simulink model "UserSteerTorque"  (Simulink 7.5)
settings: Solver=ode45  StartTime=0.0  StopTime=inf  RelTol=1e-3
libraries: CarMaker4SL x4, simulink x1
(part 2 of 2)

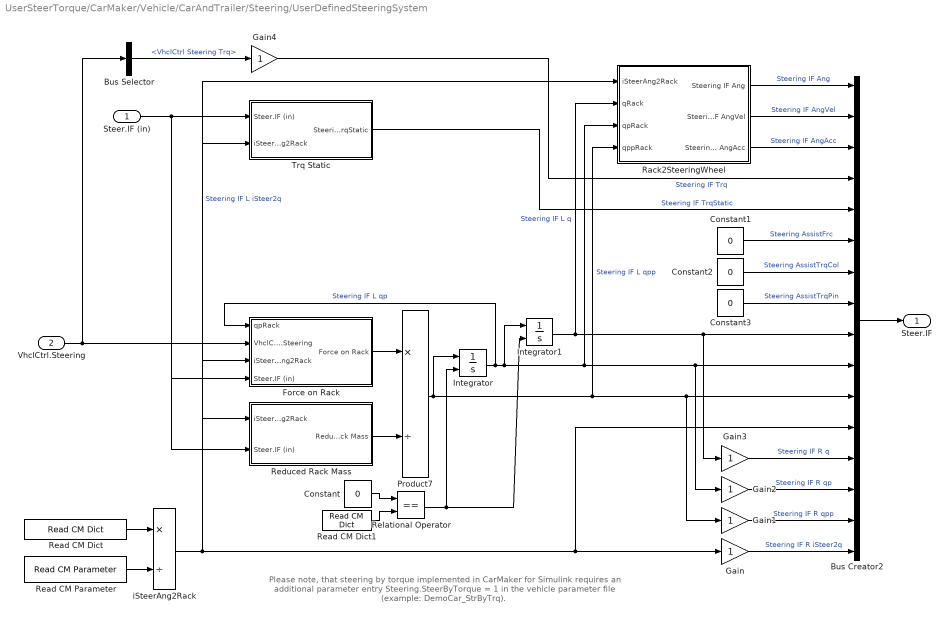
== system UserSteerTorque/CarMaker/Vehicle/CarAndTrailer/Steering/UserDefinedSteeringSystem ==
  note: Please note, that steering by torque implemented in
      | CarMaker for Simulink requires an additional parameter entry
      | Steering.SteerByTorque = 1
      | in the vehicle parameter file (example: DemoCar_StrByTrq).
  Steer.IF (in) : Inport  OutDataType=sfix(16)  OutScaling=2^0
  VhclCtrl.Steering : Inport  Port=2  OutDataType=sfix(16)  OutScaling=2^0
  Bus Creator2 : BusCreator  Inputs=16
  Bus Selector : BusSelector  OutputSignals=VhclCtrl Steering Trq
  Constant{,1..3} (4 alike) : Constant  Value=0  OutDataType=sfix(16)  OutScaling=2^0
  Force on Rack : Subsystem
  Gain{,1..4} (5 alike) : Gain  ParameterDataType=sfix(16)  ParameterScaling=2^0  OutDataType=sfix(16)  OutScaling=2^0
  Integrator : Integrator  ExternalReset=level
  Integrator1 : Integrator  ExternalReset=level
  Product7 : Product  Inputs=*/  OutDataType=sfix(16)  OutScaling=2^0  SaturateOnIntegerOverflow=on  InputSameDT=on  OutDataTypeStr=Inherit: Same as first input
  Rack2SteeringWheel : Subsystem
  Read CM Dict : CarMaker4SL/Read CM Dict  xname=Steer.Cfg.PosSign  xsync=off
  Read CM Dict1 : CarMaker4SL/Read CM Dict  xname=Time  xsync=off
  Read CM Parameter : CarMaker4SL/Read CM Parameter  xfile=Steering  xkey=Steering.Rack2StWhl  xnout=1  xdefaults=[]  xmuxed=off
  Reduced Rack Mass : Subsystem
  Relational Operator : RelationalOperator  Operator===
  Trq Static : Subsystem
  iSteerAng2Rack : Product  Inputs=*/  OutDataType=sfix(16)  OutScaling=2^0  SaturateOnIntegerOverflow=on  InputSameDT=on  OutDataTypeStr=Inherit: Same as first input
  Steer.IF : Outport  OutDataType=sfix(16)  OutScaling=2^0
  wires:
  Bus Selector/1 -> Gain4/1  "<VhclCtrl Steering Trq>"
  Gain4/1 -> Bus Creator2/4  "Steering IF Trq"
  Gain3/1 -> Bus Creator2/13  "Steering IF R q"
  Gain2/1 -> Bus Creator2/14  "Steering IF R qp"
  Gain1/1 -> Bus Creator2/15  "Steering IF R qpp"
  Gain/1 -> Bus Creator2/16  "Steering IF R iSteer2q"
  Read CM Dict/1 -> iSteerAng2Rack/1
  Read CM Parameter/1 -> iSteerAng2Rack/2
  Steer.IF (in)/1 -> Trq Static/1(Steer.IF (in)), Force on Rack/4(Steer.IF (in)), Reduced Rack Mass/2(Steer.IF (in))
  Force on Rack/1(Force on Rack) -> Product7/1
  Reduced Rack Mass/1(Reduced Rack Mass) -> Product7/2
  iSteerAng2Rack/1 -> Rack2SteeringWheel/1(iSteerAng2Rack), Trq Static/2(iSteerAng2Rack), Force on Rack/3(iSteerAng2Rack), Reduced Rack Mass/1(iSteerAng2Rack), Gain/1, Bus Creator2/12  "Steering IF L iSteer2q"
  Integrator1/1 -> Rack2SteeringWheel/2(qRack), Gain3/1, Bus Creator2/9  "Steering IF L q"
  Trq Static/1(Steering IF TrqStatic) -> Bus Creator2/5  "Steering IF TrqStatic"
  Rack2SteeringWheel/1(Steering IF Ang) -> Bus Creator2/1  "Steering IF Ang"
  Rack2SteeringWheel/2(Steering IF AngVel) -> Bus Creator2/2  "Steering IF AngVel"
  Rack2SteeringWheel/3(Steering IF AngAcc) -> Bus Creator2/3  "Steering IF AngAcc"
  VhclCtrl.Steering/1 -> Bus Selector/1, Force on Rack/2(VhclCtrl.Steering)
  Integrator/1 -> Force on Rack/1(qpRack), Rack2SteeringWheel/3(qpRack), Gain2/1, Bus Creator2/10, Integrator1/1  "Steering IF L qp"
  Product7/1 -> Rack2SteeringWheel/4(qppRack), Gain1/1, Bus Creator2/11, Integrator/1  "Steering IF L qpp"
  Relational Operator/1 -> Integrator/2, Integrator1/2
  Read CM Dict1/1 -> Relational Operator/2
  Constant/1 -> Relational Operator/1
  Bus Creator2/1 -> Steer.IF/1
  Constant1/1 -> Bus Creator2/6  "Steering AssistFrc"
  Constant2/1 -> Bus Creator2/7  "Steering AssistTrqCol"
  Constant3/1 -> Bus Creator2/8  "Steering AssistTrqPin"

== system UserSteerTorque/CarMaker/Vehicle/CarAndTrailer/Trailer/CreateBus Car.Hitch.FrcTrq ==
  In1 : Inport  OutDataType=sfix(16)  OutScaling=2^0
  Bus Creator7 : BusCreator  Inputs=6
  Demux7 : Demux  Outputs=6
  Car.Hitch.FrcTrq : Outport  OutDataType=sfix(16)  OutScaling=2^0
  wires:
  Demux7/1 -> Bus Creator7/1  "Car Hitch Frc2Car x"
  Demux7/2 -> Bus Creator7/2  "Car Hitch Frc2Car y"
  Demux7/3 -> Bus Creator7/3  "Car Hitch Frc2Car z"
  Demux7/4 -> Bus Creator7/4  "Car Hitch Trq2Car x"
  Demux7/5 -> Bus Creator7/5  "Car Hitch Trq2Car y"
  Demux7/6 -> Bus Creator7/6  "Car Hitch Trq2Car z"
  Bus Creator7/1 -> Car.Hitch.FrcTrq/1
  In1/1 -> Demux7/1

== system UserSteerTorque/CarMaker/Vehicle/CarAndTrailer/Trailer/CreateBus Vhcl.Motion ==
  In1 : Inport  OutDataType=sfix(16)  OutScaling=2^0
  Demux1 : Demux  Outputs=16
  Mux1 : Mux  Inputs=16
  Out1 : Outport  OutDataType=sfix(16)  OutScaling=2^0
  wires:
  Mux1/1 -> Out1/1
  In1/1 -> Demux1/1
  Demux1/16 -> Mux1/16  "Vhcl YawAcc"
  Demux1/15 -> Mux1/15  "Vhcl YawRate"
  Demux1/14 -> Mux1/14  "Vhcl Yaw"
  Demux1/13 -> Mux1/13  "Vhcl PitchAcc"
  Demux1/12 -> Mux1/12  "Vhcl PitchVel"
  Demux1/11 -> Mux1/11  "Vhcl Pitch"
  Demux1/10 -> Mux1/10  "Vhcl RollAcc"
  Demux1/9 -> Mux1/9  "Vhcl RollVel"
  Demux1/8 -> Mux1/8  "Vhcl Roll"
  Demux1/7 -> Mux1/7  "Vhcl Hitch_Pos z"
  Demux1/6 -> Mux1/6  "Vhcl Hitch_Pos y"
  Demux1/5 -> Mux1/5  "Vhcl Hitch_Pos x"
  Demux1/4 -> Mux1/4  "Vhcl sRoadAero"
  Demux1/3 -> Mux1/3  "Vhcl sRoad"
  Demux1/2 -> Mux1/2  "Vhcl Distance"
  Demux1/1 -> Mux1/1  "Vhcl v"

== system UserSteerTorque/CarMaker/Vehicle/CarAndTrailer/Trailer/CreateBus Vhcl.PoI ==
  In1 : Inport  OutDataType=sfix(16)  OutScaling=2^0
  Bus Creator3 : BusCreator  Inputs=18
  Demux3 : Demux  Outputs=18
  Out1 : Outport  OutDataType=sfix(16)  OutScaling=2^0
  wires:
  Demux3/1 -> Bus Creator3/1  "Vhcl PoI_Pos x"
  Bus Creator3/1 -> Out1/1
  In1/1 -> Demux3/1
  Demux3/2 -> Bus Creator3/2  "Vhcl PoI_Pos y"
  Demux3/3 -> Bus Creator3/3  "Vhcl PoI_Pos z"
  Demux3/4 -> Bus Creator3/4  "Vhcl PoI_Vel x"
  Demux3/5 -> Bus Creator3/5  "Vhcl PoI_Vel y"
  Demux3/6 -> Bus Creator3/6  "Vhcl PoI_Vel z"
  Demux3/7 -> Bus Creator3/7  "Vhcl PoI_Acc x"
  Demux3/8 -> Bus Creator3/8  "Vhcl PoI_Acc y"
  Demux3/9 -> Bus Creator3/9  "Vhcl PoI_Acc z"
  Demux3/10 -> Bus Creator3/10  "Vhcl PoI_Vel_1 x"
  Demux3/11 -> Bus Creator3/11  "Vhcl PoI_Vel_1 y"
  Demux3/12 -> Bus Creator3/12  "Vhcl PoI_Vel_1 z"
  Demux3/13 -> Bus Creator3/13  "Vhcl PoI_Acc_1 x"
  Demux3/14 -> Bus Creator3/14  "Vhcl PoI_Acc_1 y"
  Demux3/15 -> Bus Creator3/15  "Vhcl PoI_Acc_1 z"
  Demux3/16 -> Bus Creator3/16  "Vhcl PoI_GCS Long"
  Demux3/17 -> Bus Creator3/17  "Vhcl PoI_GCS Lat"
  Demux3/18 -> Bus Creator3/18  "Vhcl PoI_GCS Elev"

== system UserSteerTorque/CarMaker/Vehicle/CarAndTrailer/Trailer/CreateBus Vhcl.Steering ==
  In1 : Inport  OutDataType=sfix(16)  OutScaling=2^0
  Bus Creator3 : BusCreator
  Demux : Demux
  Out1 : Outport  OutDataType=sfix(16)  OutScaling=2^0
  wires:
  In1/1 -> Demux/1
  Demux/4 -> Bus Creator3/4  "Vhcl Steering Trq"
  Demux/2 -> Bus Creator3/2  "Vhcl Steering AngVel"
  Demux/3 -> Bus Creator3/3  "Vhcl Steering AngAcc"
  Demux/1 -> Bus Creator3/1  "Vhcl Steering Ang"
  Bus Creator3/1 -> Out1/1

== system UserSteerTorque/CarMaker/Vehicle/CarAndTrailer/Trailer/CreateBus Vhcl.Wheel.FL ==
  In1 : Inport  OutDataType=sfix(16)  OutScaling=2^0
  Bus Creator3 : BusCreator  Inputs=14
  Demux3 : Demux  Outputs=14
  Out1 : Outport  OutDataType=sfix(16)  OutScaling=2^0
  wires:
  Demux3/1 -> Bus Creator3/1  "Vhcl Wheel FL t x"
  Bus Creator3/1 -> Out1/1
  In1/1 -> Demux3/1
  Demux3/2 -> Bus Creator3/2  "Vhcl Wheel FL t y"
  Demux3/3 -> Bus Creator3/3  "Vhcl Wheel FL t z"
  Demux3/4 -> Bus Creator3/4  "Vhcl Wheel FL r_zxy x"
  Demux3/5 -> Bus Creator3/5  "Vhcl Wheel FL r_zxy y"
  Demux3/6 -> Bus Creator3/6  "Vhcl Wheel FL r_zxy z"
  Demux3/7 -> Bus Creator3/7  "Vhcl Wheel FL Fx"
  Demux3/8 -> Bus Creator3/8  "Vhcl Wheel FL Fy"
  Demux3/9 -> Bus Creator3/9  "Vhcl Wheel FL Fz"
  Demux3/10 -> Bus Creator3/10  "Vhcl Wheel FL vBelt"
  Demux3/11 -> Bus Creator3/11  "Vhcl Wheel FL LongSlip"
  Demux3/12 -> Bus Creator3/12  "Vhcl Wheel FL SideSlip"
  Demux3/13 -> Bus Creator3/13  "Vhcl Wheel FL Trq_T2W"
  Demux3/14 -> Bus Creator3/14  "Vhcl Wheel FL Trq_WhlBearing"

== system UserSteerTorque/CarMaker/Vehicle/CarAndTrailer/Trailer/CreateBus Vhcl.Wheel.FR ==
  In1 : Inport  OutDataType=sfix(16)  OutScaling=2^0
  Bus Creator3 : BusCreator  Inputs=14
  Demux3 : Demux  Outputs=14
  Out1 : Outport  OutDataType=sfix(16)  OutScaling=2^0
  wires:
  Demux3/1 -> Bus Creator3/1  "Vhcl Wheel FR t x"
  Bus Creator3/1 -> Out1/1
  In1/1 -> Demux3/1
  Demux3/2 -> Bus Creator3/2  "Vhcl Wheel FR t y"
  Demux3/3 -> Bus Creator3/3  "Vhcl Wheel FR t z"
  Demux3/4 -> Bus Creator3/4  "Vhcl Wheel FR r_zxy x"
  Demux3/5 -> Bus Creator3/5  "Vhcl Wheel FR r_zxy y"
  Demux3/6 -> Bus Creator3/6  "Vhcl Wheel FR r_zxy z"
  Demux3/7 -> Bus Creator3/7  "Vhcl Wheel FR Fx"
  Demux3/8 -> Bus Creator3/8  "Vhcl Wheel FR Fy"
  Demux3/9 -> Bus Creator3/9  "Vhcl Wheel FR Fz"
  Demux3/10 -> Bus Creator3/10  "Vhcl Wheel FR vBelt"
  Demux3/11 -> Bus Creator3/11  "Vhcl Wheel FR LongSlip"
  Demux3/12 -> Bus Creator3/12  "Vhcl Wheel FR SideSlip"
  Demux3/13 -> Bus Creator3/13  "Vhcl Wheel FR Trq_T2W"
  Demux3/14 -> Bus Creator3/14  "Vhcl Wheel FR Trq_WhlBearing"

== system UserSteerTorque/CarMaker/Vehicle/CarAndTrailer/Trailer/CreateBus Vhcl.Wheel.RL ==
  In1 : Inport  OutDataType=sfix(16)  OutScaling=2^0
  Bus Creator3 : BusCreator  Inputs=14
  Demux3 : Demux  Outputs=14
  Out1 : Outport  OutDataType=sfix(16)  OutScaling=2^0
  wires:
  Demux3/1 -> Bus Creator3/1  "Vhcl Wheel RL t x"
  Bus Creator3/1 -> Out1/1
  In1/1 -> Demux3/1
  Demux3/2 -> Bus Creator3/2  "Vhcl Wheel RL t y"
  Demux3/3 -> Bus Creator3/3  "Vhcl Wheel RL t z"
  Demux3/4 -> Bus Creator3/4  "Vhcl Wheel RL r_zxy x"
  Demux3/5 -> Bus Creator3/5  "Vhcl Wheel RL r_zxy y"
  Demux3/6 -> Bus Creator3/6  "Vhcl Wheel RL r_zxy z"
  Demux3/7 -> Bus Creator3/7  "Vhcl Wheel RL Fx"
  Demux3/8 -> Bus Creator3/8  "Vhcl Wheel RL Fy"
  Demux3/9 -> Bus Creator3/9  "Vhcl Wheel RL Fz"
  Demux3/10 -> Bus Creator3/10  "Vhcl Wheel RL vBelt"
  Demux3/11 -> Bus Creator3/11  "Vhcl Wheel RL LongSlip"
  Demux3/12 -> Bus Creator3/12  "Vhcl Wheel RL SideSlip"
  Demux3/13 -> Bus Creator3/13  "Vhcl Wheel RL Trq_T2W"
  Demux3/14 -> Bus Creator3/14  "Vhcl Wheel RL Trq_WhlBearing"

== system UserSteerTorque/CarMaker/Vehicle/CarAndTrailer/Trailer/CreateBus Vhcl.Wheel.RR ==
  In1 : Inport  OutDataType=sfix(16)  OutScaling=2^0
  Bus Creator3 : BusCreator  Inputs=14
  Demux3 : Demux  Outputs=14
  Out1 : Outport  OutDataType=sfix(16)  OutScaling=2^0
  wires:
  Demux3/1 -> Bus Creator3/1  "Vhcl Wheel RR t x"
  Bus Creator3/1 -> Out1/1
  In1/1 -> Demux3/1
  Demux3/2 -> Bus Creator3/2  "Vhcl Wheel RR t y"
  Demux3/3 -> Bus Creator3/3  "Vhcl Wheel RR t z"
  Demux3/4 -> Bus Creator3/4  "Vhcl Wheel RR r_zxy x"
  Demux3/5 -> Bus Creator3/5  "Vhcl Wheel RR r_zxy y"
  Demux3/6 -> Bus Creator3/6  "Vhcl Wheel RR r_zxy z"
  Demux3/7 -> Bus Creator3/7  "Vhcl Wheel RR Fx"
  Demux3/8 -> Bus Creator3/8  "Vhcl Wheel RR Fy"
  Demux3/9 -> Bus Creator3/9  "Vhcl Wheel RR Fz"
  Demux3/10 -> Bus Creator3/10  "Vhcl Wheel RR vBelt"
  Demux3/11 -> Bus Creator3/11  "Vhcl Wheel RR LongSlip"
  Demux3/12 -> Bus Creator3/12  "Vhcl Wheel RR SideSlip"
  Demux3/13 -> Bus Creator3/13  "Vhcl Wheel RR Trq_T2W"
  Demux3/14 -> Bus Creator3/14  "Vhcl Wheel RR Trq_WhlBearing"

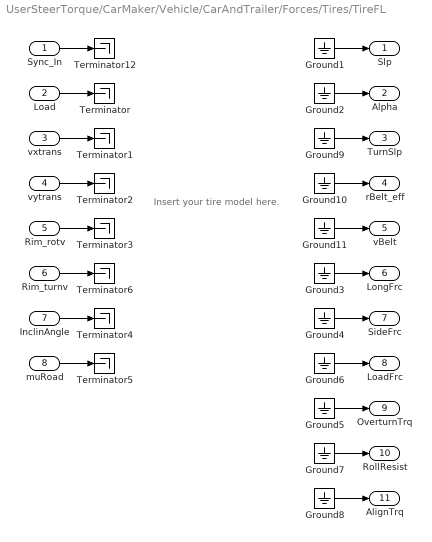
== system UserSteerTorque/CarMaker/Vehicle/CarAndTrailer/Forces/Tires/TireFL ==
  note: Insert your tire model here.
  Sync_In : Inport  OutDataType=sfix(16)  OutScaling=2^0
  Load : Inport  Port=2  OutDataType=sfix(16)  OutScaling=2^0
  vxtrans : Inport  Port=3  OutDataType=sfix(16)  OutScaling=2^0
  vytrans : Inport  Port=4  OutDataType=sfix(16)  OutScaling=2^0
  Rim_rotv : Inport  Port=5  OutDataType=sfix(16)  OutScaling=2^0
  Rim_turnv : Inport  Port=6  OutDataType=sfix(16)  OutScaling=2^0
  InclinAngle : Inport  Port=7  OutDataType=sfix(16)  OutScaling=2^0
  muRoad : Inport  Port=8  OutDataType=sfix(16)  OutScaling=2^0
  Ground{1..11} (11 alike) : Ground
  Terminator{,1..6,12} (8 alike) : Terminator
  Slp : Outport  OutDataType=sfix(16)  OutScaling=2^0
  Alpha : Outport  Port=2  OutDataType=sfix(16)  OutScaling=2^0
  TurnSlp : Outport  Port=3  OutDataType=sfix(16)  OutScaling=2^0
  rBelt_eff : Outport  Port=4  OutDataType=sfix(16)  OutScaling=2^0
  vBelt : Outport  Port=5  OutDataType=sfix(16)  OutScaling=2^0
  LongFrc : Outport  Port=6  OutDataType=sfix(16)  OutScaling=2^0
  SideFrc : Outport  Port=7  OutDataType=sfix(16)  OutScaling=2^0
  LoadFrc : Outport  Port=8  OutDataType=sfix(16)  OutScaling=2^0
  OverturnTrq : Outport  Port=9  OutDataType=sfix(16)  OutScaling=2^0
  RollResist : Outport  Port=10  OutDataType=sfix(16)  OutScaling=2^0
  AlignTrq : Outport  Port=11  OutDataType=sfix(16)  OutScaling=2^0
  wires:
  Ground8/1 -> AlignTrq/1
  Ground7/1 -> RollResist/1
  Ground6/1 -> LoadFrc/1
  Ground1/1 -> Slp/1
  Load/1 -> Terminator/1
  muRoad/1 -> Terminator5/1
  InclinAngle/1 -> Terminator4/1
  Rim_rotv/1 -> Terminator3/1
  vytrans/1 -> Terminator2/1
  vxtrans/1 -> Terminator1/1
  Ground5/1 -> OverturnTrq/1
  Ground4/1 -> SideFrc/1
  Ground3/1 -> LongFrc/1
  Ground2/1 -> Alpha/1
  Sync_In/1 -> Terminator12/1
  Rim_turnv/1 -> Terminator6/1
  Ground9/1 -> TurnSlp/1
  Ground10/1 -> rBelt_eff/1
  Ground11/1 -> vBelt/1

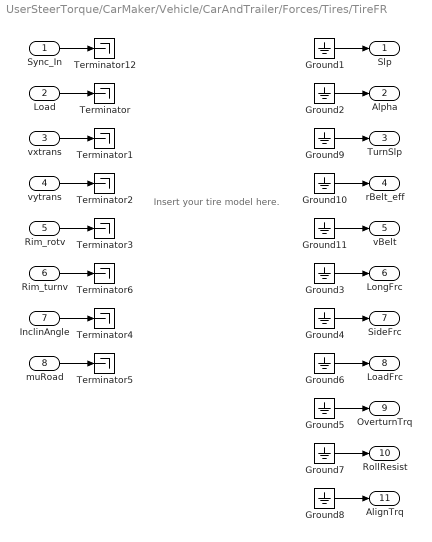
== system UserSteerTorque/CarMaker/Vehicle/CarAndTrailer/Forces/Tires/TireFR ==
  note: Insert your tire model here.
  Sync_In : Inport  OutDataType=sfix(16)  OutScaling=2^0
  Load : Inport  Port=2  OutDataType=sfix(16)  OutScaling=2^0
  vxtrans : Inport  Port=3  OutDataType=sfix(16)  OutScaling=2^0
  vytrans : Inport  Port=4  OutDataType=sfix(16)  OutScaling=2^0
  Rim_rotv : Inport  Port=5  OutDataType=sfix(16)  OutScaling=2^0
  Rim_turnv : Inport  Port=6  OutDataType=sfix(16)  OutScaling=2^0
  InclinAngle : Inport  Port=7  OutDataType=sfix(16)  OutScaling=2^0
  muRoad : Inport  Port=8  OutDataType=sfix(16)  OutScaling=2^0
  Ground{1..11} (11 alike) : Ground
  Terminator{,1..6,12} (8 alike) : Terminator
  Slp : Outport  OutDataType=sfix(16)  OutScaling=2^0
  Alpha : Outport  Port=2  OutDataType=sfix(16)  OutScaling=2^0
  TurnSlp : Outport  Port=3  OutDataType=sfix(16)  OutScaling=2^0
  rBelt_eff : Outport  Port=4  OutDataType=sfix(16)  OutScaling=2^0
  vBelt : Outport  Port=5  OutDataType=sfix(16)  OutScaling=2^0
  LongFrc : Outport  Port=6  OutDataType=sfix(16)  OutScaling=2^0
  SideFrc : Outport  Port=7  OutDataType=sfix(16)  OutScaling=2^0
  LoadFrc : Outport  Port=8  OutDataType=sfix(16)  OutScaling=2^0
  OverturnTrq : Outport  Port=9  OutDataType=sfix(16)  OutScaling=2^0
  RollResist : Outport  Port=10  OutDataType=sfix(16)  OutScaling=2^0
  AlignTrq : Outport  Port=11  OutDataType=sfix(16)  OutScaling=2^0
  wires:
  Ground8/1 -> AlignTrq/1
  Ground7/1 -> RollResist/1
  Ground6/1 -> LoadFrc/1
  Ground1/1 -> Slp/1
  Load/1 -> Terminator/1
  muRoad/1 -> Terminator5/1
  InclinAngle/1 -> Terminator4/1
  Rim_rotv/1 -> Terminator3/1
  vytrans/1 -> Terminator2/1
  vxtrans/1 -> Terminator1/1
  Ground5/1 -> OverturnTrq/1
  Ground4/1 -> SideFrc/1
  Ground3/1 -> LongFrc/1
  Ground2/1 -> Alpha/1
  Sync_In/1 -> Terminator12/1
  Rim_turnv/1 -> Terminator6/1
  Ground9/1 -> TurnSlp/1
  Ground10/1 -> rBelt_eff/1
  Ground11/1 -> vBelt/1

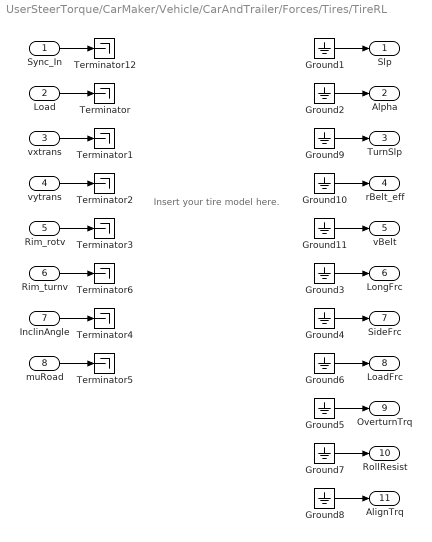
== system UserSteerTorque/CarMaker/Vehicle/CarAndTrailer/Forces/Tires/TireRL ==
  note: Insert your tire model here.
  Sync_In : Inport  OutDataType=sfix(16)  OutScaling=2^0
  Load : Inport  Port=2  OutDataType=sfix(16)  OutScaling=2^0
  vxtrans : Inport  Port=3  OutDataType=sfix(16)  OutScaling=2^0
  vytrans : Inport  Port=4  OutDataType=sfix(16)  OutScaling=2^0
  Rim_rotv : Inport  Port=5  OutDataType=sfix(16)  OutScaling=2^0
  Rim_turnv : Inport  Port=6  OutDataType=sfix(16)  OutScaling=2^0
  InclinAngle : Inport  Port=7  OutDataType=sfix(16)  OutScaling=2^0
  muRoad : Inport  Port=8  OutDataType=sfix(16)  OutScaling=2^0
  Ground{1..11} (11 alike) : Ground
  Terminator{,1..6,12} (8 alike) : Terminator
  Slp : Outport  OutDataType=sfix(16)  OutScaling=2^0
  Alpha : Outport  Port=2  OutDataType=sfix(16)  OutScaling=2^0
  TurnSlp : Outport  Port=3  OutDataType=sfix(16)  OutScaling=2^0
  rBelt_eff : Outport  Port=4  OutDataType=sfix(16)  OutScaling=2^0
  vBelt : Outport  Port=5  OutDataType=sfix(16)  OutScaling=2^0
  LongFrc : Outport  Port=6  OutDataType=sfix(16)  OutScaling=2^0
  SideFrc : Outport  Port=7  OutDataType=sfix(16)  OutScaling=2^0
  LoadFrc : Outport  Port=8  OutDataType=sfix(16)  OutScaling=2^0
  OverturnTrq : Outport  Port=9  OutDataType=sfix(16)  OutScaling=2^0
  RollResist : Outport  Port=10  OutDataType=sfix(16)  OutScaling=2^0
  AlignTrq : Outport  Port=11  OutDataType=sfix(16)  OutScaling=2^0
  wires:
  Ground8/1 -> AlignTrq/1
  Ground7/1 -> RollResist/1
  Ground6/1 -> LoadFrc/1
  Ground1/1 -> Slp/1
  Load/1 -> Terminator/1
  muRoad/1 -> Terminator5/1
  InclinAngle/1 -> Terminator4/1
  Rim_rotv/1 -> Terminator3/1
  vytrans/1 -> Terminator2/1
  vxtrans/1 -> Terminator1/1
  Ground5/1 -> OverturnTrq/1
  Ground4/1 -> SideFrc/1
  Ground3/1 -> LongFrc/1
  Ground2/1 -> Alpha/1
  Sync_In/1 -> Terminator12/1
  Rim_turnv/1 -> Terminator6/1
  Ground9/1 -> TurnSlp/1
  Ground10/1 -> rBelt_eff/1
  Ground11/1 -> vBelt/1

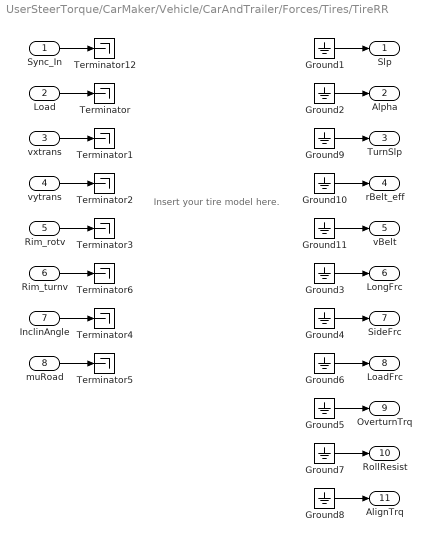
== system UserSteerTorque/CarMaker/Vehicle/CarAndTrailer/Forces/Tires/TireRR ==
  note: Insert your tire model here.
  Sync_In : Inport  OutDataType=sfix(16)  OutScaling=2^0
  Load : Inport  Port=2  OutDataType=sfix(16)  OutScaling=2^0
  vxtrans : Inport  Port=3  OutDataType=sfix(16)  OutScaling=2^0
  vytrans : Inport  Port=4  OutDataType=sfix(16)  OutScaling=2^0
  Rim_rotv : Inport  Port=5  OutDataType=sfix(16)  OutScaling=2^0
  Rim_turnv : Inport  Port=6  OutDataType=sfix(16)  OutScaling=2^0
  InclinAngle : Inport  Port=7  OutDataType=sfix(16)  OutScaling=2^0
  muRoad : Inport  Port=8  OutDataType=sfix(16)  OutScaling=2^0
  Ground{1..11} (11 alike) : Ground
  Terminator{,1..6,12} (8 alike) : Terminator
  Slp : Outport  OutDataType=sfix(16)  OutScaling=2^0
  Alpha : Outport  Port=2  OutDataType=sfix(16)  OutScaling=2^0
  TurnSlp : Outport  Port=3  OutDataType=sfix(16)  OutScaling=2^0
  rBelt_eff : Outport  Port=4  OutDataType=sfix(16)  OutScaling=2^0
  vBelt : Outport  Port=5  OutDataType=sfix(16)  OutScaling=2^0
  LongFrc : Outport  Port=6  OutDataType=sfix(16)  OutScaling=2^0
  SideFrc : Outport  Port=7  OutDataType=sfix(16)  OutScaling=2^0
  LoadFrc : Outport  Port=8  OutDataType=sfix(16)  OutScaling=2^0
  OverturnTrq : Outport  Port=9  OutDataType=sfix(16)  OutScaling=2^0
  RollResist : Outport  Port=10  OutDataType=sfix(16)  OutScaling=2^0
  AlignTrq : Outport  Port=11  OutDataType=sfix(16)  OutScaling=2^0
  wires:
  Ground8/1 -> AlignTrq/1
  Ground7/1 -> RollResist/1
  Ground6/1 -> LoadFrc/1
  Ground1/1 -> Slp/1
  Load/1 -> Terminator/1
  muRoad/1 -> Terminator5/1
  InclinAngle/1 -> Terminator4/1
  Rim_rotv/1 -> Terminator3/1
  vytrans/1 -> Terminator2/1
  vxtrans/1 -> Terminator1/1
  Ground5/1 -> OverturnTrq/1
  Ground4/1 -> SideFrc/1
  Ground3/1 -> LongFrc/1
  Ground2/1 -> Alpha/1
  Sync_In/1 -> Terminator12/1
  Rim_turnv/1 -> Terminator6/1
  Ground9/1 -> TurnSlp/1
  Ground10/1 -> rBelt_eff/1
  Ground11/1 -> vBelt/1

== system UserSteerTorque/CarMaker/Vehicle/CarAndTrailer/Steering/UserDefinedSteeringSystem/Force on Rack ==
  qpRack : Inport  OutDataType=sfix(16)  OutScaling=2^0
  VhclCtrl.Steering : Inport  Port=2  OutDataType=sfix(16)  OutScaling=2^0
  iSteerAng2Rack : Inport  Port=3  OutDataType=sfix(16)  OutScaling=2^0
  Steer.IF (in) : Inport  Port=4  OutDataType=sfix(16)  OutScaling=2^0
  Abs : Abs  SaturateOnIntegerOverflow=on
  Bus Selector : BusSelector  OutputSignals=VhclCtrl Steering Trq
  Bus Selector1 : BusSelector  OutputSignals=Steering IF L Frc,Steering IF R Frc
  Product10 : Product  Inputs=*/*  OutDataType=sfix(16)  OutScaling=2^0  SaturateOnIntegerOverflow=on  InputSameDT=on  OutDataTypeStr=Inherit: Same as first input
  Product11 : Product  Inputs=*/  OutDataType=sfix(16)  OutScaling=2^0  SaturateOnIntegerOverflow=on  InputSameDT=on  OutDataTypeStr=Inherit: Same as first input
  Rack Damping : Constant  Value=200  OutDataType=sfix(16)  OutScaling=2^0
  Sum2 : Sum  Inputs=+++-  OutDataType=sfix(16)  OutScaling=2^0  SaturateOnIntegerOverflow=on  InputSameDT=on  OutDataTypeStr=Inherit: Same as first input
  Force on Rack : Outport  OutDataType=sfix(16)  OutScaling=2^0
  wires:
  Product11/1 -> Sum2/3  "TrqDriver2Rack"
  VhclCtrl.Steering/1 -> Bus Selector/1
  Bus Selector/1 -> Product11/1  "<VhclCtrl Steering Trq>"
  Bus Selector1/2 -> Sum2/2  "<Steering IF R Frc>"
  Bus Selector1/1 -> Sum2/1  "<Steering IF L Frc>"
  Steer.IF (in)/1 -> Bus Selector1/1
  Sum2/1 -> Force on Rack/1
  iSteerAng2Rack/1 -> Product11/2, Abs/1
  qpRack/1 -> Product10/3
  Abs/1 -> Product10/2
  Product10/1 -> Sum2/4  "Damping Force"
  Rack Damping/1 -> Product10/1

== system UserSteerTorque/CarMaker/Vehicle/CarAndTrailer/Steering/UserDefinedSteeringSystem/Rack2SteeringWheel ==
  iSteerAng2Rack : Inport  OutDataType=sfix(16)  OutScaling=2^0
  qRack : Inport  Port=2  OutDataType=sfix(16)  OutScaling=2^0
  qpRack : Inport  Port=3  OutDataType=sfix(16)  OutScaling=2^0
  qppRack : Inport  Port=4  OutDataType=sfix(16)  OutScaling=2^0
  Product1 : Product  Inputs=*/  OutDataType=sfix(16)  OutScaling=2^0  SaturateOnIntegerOverflow=on  InputSameDT=on  OutDataTypeStr=Inherit: Same as first input
  Product2 : Product  Inputs=*/  OutDataType=sfix(16)  OutScaling=2^0  SaturateOnIntegerOverflow=on  InputSameDT=on  OutDataTypeStr=Inherit: Same as first input
  Product3 : Product  Inputs=*/  OutDataType=sfix(16)  OutScaling=2^0  SaturateOnIntegerOverflow=on  InputSameDT=on  OutDataTypeStr=Inherit: Same as first input
  Steering IF Ang : Outport  OutDataType=sfix(16)  OutScaling=2^0
  Steering IF AngVel : Outport  Port=2  OutDataType=sfix(16)  OutScaling=2^0
  Steering IF AngAcc : Outport  Port=3  OutDataType=sfix(16)  OutScaling=2^0
  wires:
  iSteerAng2Rack/1 -> Product3/2, Product1/2, Product2/2
  qppRack/1 -> Product3/1
  qpRack/1 -> Product2/1
  qRack/1 -> Product1/1
  Product3/1 -> Steering IF AngAcc/1
  Product2/1 -> Steering IF AngVel/1
  Product1/1 -> Steering IF Ang/1

== system UserSteerTorque/CarMaker/Vehicle/CarAndTrailer/Steering/UserDefinedSteeringSystem/Reduced Rack Mass ==
  iSteerAng2Rack : Inport  OutDataType=sfix(16)  OutScaling=2^0
  Steer.IF (in) : Inport  Port=2  OutDataType=sfix(16)  OutScaling=2^0
  Bus Selector1 : BusSelector  OutputSignals=Steering IF L Inert,Steering IF R Inert
  Product8 : Product  Inputs=*/  OutDataType=sfix(16)  OutScaling=2^0  SaturateOnIntegerOverflow=on  InputSameDT=on  OutDataTypeStr=Inherit: Same as first input
  Product9 : Product  Inputs=**  OutDataType=sfix(16)  OutScaling=2^0  SaturateOnIntegerOverflow=on  InputSameDT=on  OutDataTypeStr=Inherit: Same as first input
  SteeringWheel.Irot [km*m^2] : Constant  Value=0.03  OutDataType=sfix(16)  OutScaling=2^0
  Sum1 : Sum  Inputs=+++  OutDataType=sfix(16)  OutScaling=2^0  SaturateOnIntegerOverflow=on  InputSameDT=on  OutDataTypeStr=Inherit: Same as first input
  Reduced Rack Mass : Outport  OutDataType=sfix(16)  OutScaling=2^0
  wires:
  iSteerAng2Rack/1 -> Product9/2, Product9/1
  Product9/1 -> Product8/2
  Product8/1 -> Sum1/1
  Bus Selector1/2 -> Sum1/3  "<Steering IF R Inert>"
  Bus Selector1/1 -> Sum1/2  "<Steering IF L Inert>"
  Steer.IF (in)/1 -> Bus Selector1/1
  Sum1/1 -> Reduced Rack Mass/1
  SteeringWheel.Irot [km*m^2]/1 -> Product8/1

== system UserSteerTorque/CarMaker/Vehicle/CarAndTrailer/Steering/UserDefinedSteeringSystem/Trq Static ==
  Steer.IF (in) : Inport  OutDataType=sfix(16)  OutScaling=2^0
  iSteerAng2Rack : Inport  Port=2  OutDataType=sfix(16)  OutScaling=2^0
  Bus Selector1 : BusSelector  OutputSignals=Steering IF L Frc,Steering IF R Frc
  Product6 : Product  OutDataType=sfix(16)  OutScaling=2^0  SaturateOnIntegerOverflow=on  InputSameDT=on  OutDataTypeStr=Inherit: Same as first input
  Sum : Sum  Inputs=--  OutDataType=sfix(16)  OutScaling=2^0  SaturateOnIntegerOverflow=on  InputSameDT=on  OutDataTypeStr=Inherit: Same as first input
  Steering IF TrqStatic : Outport  OutDataType=sfix(16)  OutScaling=2^0
  wires:
  Product6/1 -> Steering IF TrqStatic/1
  iSteerAng2Rack/1 -> Product6/2
  Steer.IF (in)/1 -> Bus Selector1/1
  Bus Selector1/2 -> Sum/2  "<Steering IF R Frc>"
  Sum/1 -> Product6/1
  Bus Selector1/1 -> Sum/1  "<Steering IF L Frc>"
